simulink model "linearni_kyvadlo"  (R2017b)
settings: Solver=VariableStepAuto  StartTime=0.0  StopTime=10  MaxStep=0.015  RelTol=1e-3
settings Model: Creator=ladislav  LastModifiedBy=ladislav

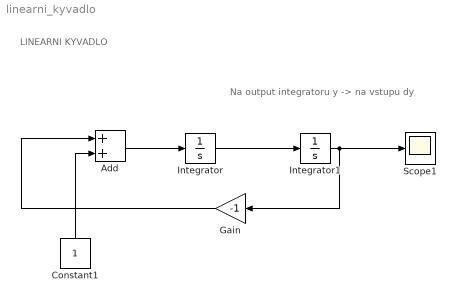
== system linearni_kyvadlo ==
  note: LINEARNI KYVADLO
  note: Na output integratoru y -> na vstupu dy
  Add : Sum
  Constant1 : Constant
  Gain : Gain  Gain=-1
  Integrator : Integrator
  Integrator1 : Integrator  InitialCondition=2
  Scope1 : Scope
  wires:
  Integrator1/1 -> Scope1/1, Gain/1
  Integrator/1 -> Integrator1/1
  Add/1 -> Integrator/1
  Constant1/1 -> Add/2
  Gain/1 -> Add/1
